simulink model "Control_PWM_Pulmon_borra2"  (R2018a)
settings: Solver=ode45  StartTime=0.0  StopTime=5  FixedStep=5.0E-5  RelTol=1e-3
libraries: simulink x2, pePwmGenerator x1
settings Model: Creator=Ruben  LastModifiedBy=Ruben
settings SolverCC: AlgebraicLoopSolver=LineSearch

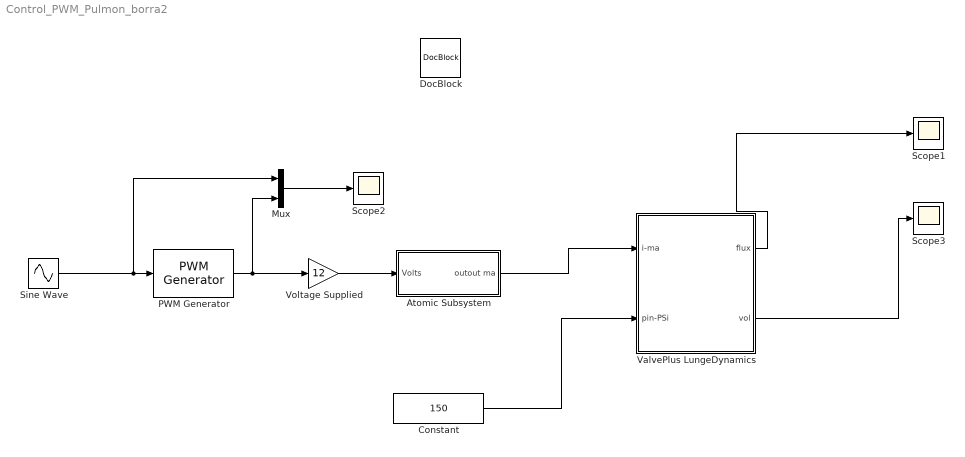
== system Control_PWM_Pulmon_borra2 ==
  Atomic Subsystem : Subsystem  TreatAsAtomicUnit=on
  Constant : Constant  Value=150
  DocBlock : simulink/Model-Wide Utilities/DocBlock  DocumentType=Text
      content=|
      | %mechanical partvalve modeling as Flux=k*i*delta P(static_Gain/(Ts+1))
      | %k=
  Mux : Mux  Inputs=2
  PWM Generator : pePwmGenerator/PWM Generator  CarrCount=Up  Tper=0.1  Ts=5e-5
  Scope1 : Scope
  Scope2 : Scope
  Scope3 : Scope
  Sine Wave : Sin  Amplitude=.5  Bias=.5  Frequency=30  SampleTime=0
  ValvePlus LungeDynamics : Subsystem
  Voltage Supplied : Gain  Gain=12
  wires:
  Sine Wave/1 -> Mux/1, PWM Generator/1
  PWM Generator/1 -> Mux/2, Voltage Supplied/1
  Mux/1 -> Scope2/1
  Voltage Supplied/1 -> Atomic Subsystem/1("Volts ")
  Atomic Subsystem/1(outout ma) -> ValvePlus LungeDynamics/1("i-ma ")
  Constant/1 -> ValvePlus LungeDynamics/2(pin-PSi)
  ValvePlus LungeDynamics/1(flux) -> Scope1/1
  ValvePlus LungeDynamics/2(vol) -> Scope3/1

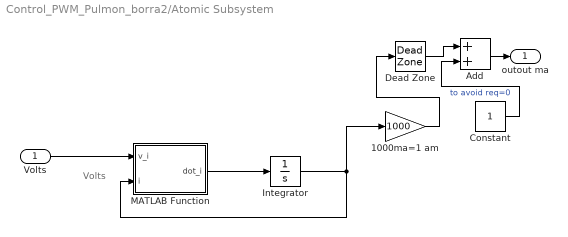
== system Control_PWM_Pulmon_borra2/Atomic Subsystem ==
  note: Volts
  "Volts " : Inport
  1000ma=1 am : Gain  Gain=1000
  Add : Sum
  Constant : Constant
  Dead Zone : DeadZone  LowerValue=0  UpperValue=250  SaturateOnIntegerOverflow=on
  Integrator : Integrator
  MATLAB Function : MATLAB Function  TreatAsAtomicUnit=on
  outout ma : Outport
  wires:
  Integrator/1 -> MATLAB Function/2(i), 1000ma=1 am/1
  MATLAB Function/1(dot_i) -> Integrator/1
  "Volts "/1 -> MATLAB Function/1(v_i)
  1000ma=1 am/1 -> Dead Zone/1
  Add/1 -> outout ma/1
  Dead Zone/1 -> Add/1
  Constant/1 -> Add/2  "to avoid req=0"

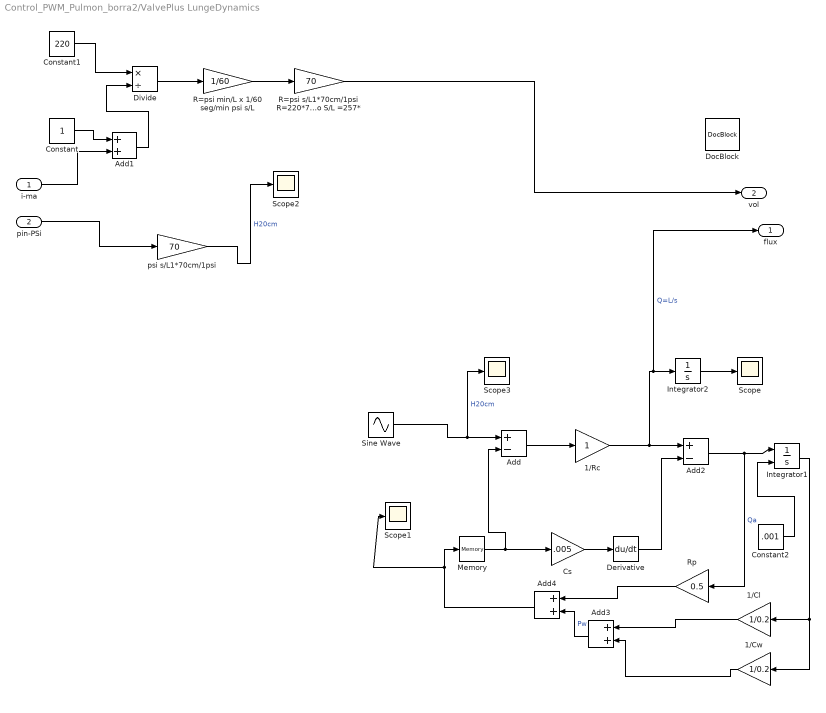
== system Control_PWM_Pulmon_borra2/ValvePlus LungeDynamics ==
  "i-ma " : Inport
  pin-PSi : Inport  Port=2
  1/Cl : Gain  Gain=1/0.2
  1/Cw : Gain  Gain=1/0.2
  1/Rc : Gain
  Add : Sum  Inputs=+-
  Add1 : Sum
  Add2 : Sum  Inputs=+-
  Add3 : Sum
  Add4 : Sum
  Constant : Constant
  Constant1 : Constant  Value=220
  Constant2 : Constant  Value=.001
  Cs : Gain  Gain=.005
  Derivative : Derivative
  Divide : Product  Inputs=*/
  DocBlock : simulink/Model-Wide Utilities/DocBlock  DocumentType=Text
      content=|
      | flux=k*I*deltaP
      |  delay = 1/(Ts+1)
      |
      | k=delta flux/ delta i % de tablas aprox 20/100
      | T=L/R  L=0.063
      | R=2
      | dead zone =250 promedio
      | %flux slpm
      | Delta P en PSI
  Integrator1 : Integrator  InitialConditionSource=external
  Integrator2 : Integrator
  Memory : Memory  InheritSampleTime=on  LinearizeMemory=on  LinearizeAsDelay=on
  R=psi min/L x 1/60 seg/min psi s/L : Gain  Gain=1/60
  R=psi s/L1*70cm/1psi R=220*70/60 cmH2o S/L =257* : Gain  Gain=70
  Rp : Gain  Gain=0.5
  Scope{,1..3} (4 alike) : Scope
  Sine Wave : Sin  Amplitude=2.5  Frequency=1.57  SampleTime=0
  "psi s/L1*70cm/1psi " : Gain  Gain=70
  flux : Outport
  vol : Outport  Port=2
  wires:
  pin-PSi/1 -> "psi s/L1*70cm/1psi "/1
  "i-ma "/1 -> Add1/2
  Constant/1 -> Add1/1
  Constant1/1 -> Divide/1
  Add1/1 -> Divide/2
  Divide/1 -> R=psi min/L x 1/60 seg/min psi s/L/1
  R=psi min/L x 1/60 seg/min psi s/L/1 -> R=psi s/L1*70cm/1psi R=220*70/60 cmH2o S/L =257*/1
  "psi s/L1*70cm/1psi "/1 -> Scope2/1  "H20cm"
  R=psi s/L1*70cm/1psi R=220*70/60 cmH2o S/L =257*/1 -> vol/1
  1/Cw/1 -> Add3/2
  Integrator2/1 -> Scope/1
  Add2/1 -> Rp/1, Integrator1/1  "Qa"
  Derivative/1 -> Add2/2
  Cs/1 -> Derivative/1
  Memory/1 -> Add/2, Cs/1
  Sine Wave/1 -> Scope3/1, Add/1  "H20cm"
  1/Rc/1 -> flux/1, Integrator2/1, Add2/1  "Q=L/s"
  Add/1 -> 1/Rc/1
  Integrator1/1 -> 1/Cw/1, 1/Cl/1
  1/Cl/1 -> Add3/1
  Rp/1 -> Add4/1
  Add3/1 -> Add4/2  "Pw"
  Add4/1 -> Scope1/1, Memory/1
  Constant2/1 -> Integrator1/2

== matlab function Control_PWM_Pulmon_borra2/Atomic Subsystem/MATLAB Function ==
  data: v_i input; dot_i output; i input
function dot_i = fcn(v_i,i)
R=20; % R igual a 2 ohm
L=.063 ;% L aprox 63mh
dot_i = (1/L)*(v_i-R*i);
